simulink model "MCLV_V2_33EP256MC506_LongHurstMotor_sensored_V2_R2014b"  (Simulink 8.4)
settings: Solver=FixedStepDiscrete  StartTime=0.0  StopTime=inf  FixedStep=.01  RelTol=1e-3
undefined symbols (not defined in the file or in its folder): A4, A8, B15, B9, C5, C6, D5, D8, F1, Max, MaxPer, ms, P20, P24, P41, P47, P53, P54, P97, Pin, PWMmax, Resol, us
libraries: MCHP_Blockset x20, simulink x4
(part 2 of 2)

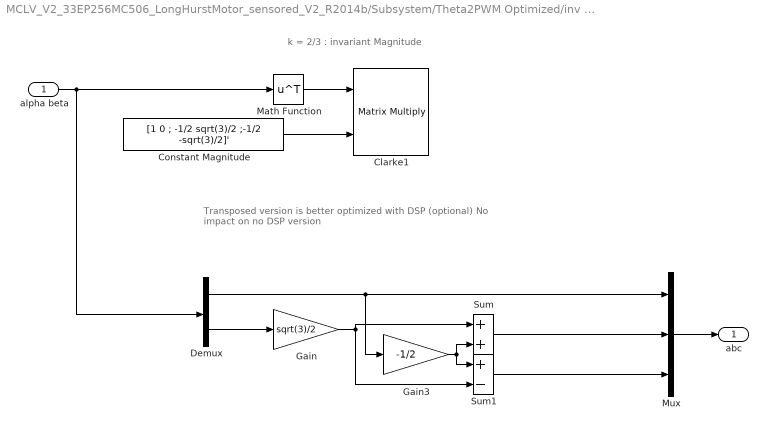
== system MCLV_V2_33EP256MC506_LongHurstMotor_sensored_V2_R2014b/Subsystem/Theta2PWM Optimized/inv Clark ==
  note: k = 2/3 : invariant Magnitude
  note: Transposed version is better optimized with DSP (optional)
      | No impact on no DSP version
  alpha beta : Inport
  Clarke1 : Product  Multiplication=Matrix(*)  RndMeth=Convergent  OutDataTypeStr=Inherit: Same as first input
  Constant Magnitude : Constant  Value=[1 0 ; -1/2 sqrt(3)/2 ;-1/2 -sqrt(3)/2]'  OutDataTypeStr=Inherit: Inherit via back propagation  SampleTime=-1
  Demux : Demux  Outputs=2
  Gain : Gain  Gain=sqrt(3)/2  OutDataTypeStr=Inherit: Same as input
  Gain3 : Gain  Gain=-1/2  RndMeth=Simplest  OutDataTypeStr=Inherit: Same as input
  Math Function : Math  Operator=transpose  SaturateOnIntegerOverflow=on
  Mux : Mux  Inputs=3
  Sum : Sum  RndMeth=Simplest  OutDataTypeStr=Inherit: Same as first input
  Sum1 : Sum  Inputs=+-  RndMeth=Simplest  OutDataTypeStr=Inherit: Same as first input
  abc : Outport
  wires:
  Gain3/1 -> Sum/2, Sum1/1
  Sum1/1 -> Mux/3
  Sum/1 -> Mux/2
  Gain/1 -> Sum1/2, Sum/1
  Demux/2 -> Gain/1
  Demux/1 -> Mux/1, Gain3/1
  Math Function/1 -> Clarke1/1
  alpha beta/1 -> Math Function/1, Demux/1
  Constant Magnitude/1 -> Clarke1/2
  Mux/1 -> abc/1

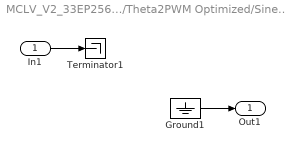
== system MCLV_V2_33EP256MC506_LongHurstMotor_sensored_V2_R2014b/Subsystem/Theta2PWM Optimized/Sine Simpler/Look-Up Table (sin) ==
  In1 : Inport
  Ground1 : Ground
  Terminator1 : Terminator
  Out1 : Outport
  wires:
  Ground1/1 -> Out1/1
  In1/1 -> Terminator1/1

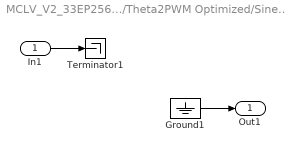
== system MCLV_V2_33EP256MC506_LongHurstMotor_sensored_V2_R2014b/Subsystem/Theta2PWM Optimized/Sine Simpler/Look-Up Table (sin)1 ==
  In1 : Inport
  Ground1 : Ground
  Terminator1 : Terminator
  Out1 : Outport
  wires:
  Ground1/1 -> Out1/1
  In1/1 -> Terminator1/1
